simulink model "Exp3_BPSK_mod_demod"  (R2020b)
settings: Solver=VariableStepAuto  StartTime=0.0  StopTime=10.0  RelTol=1e-3
libraries: simulink x3, dspsigops x2, dspstat3 x1, commrandsrc3 x1
settings Model: Creator=Mohit Akhouri  LastModifiedBy=Mohit Akhouri

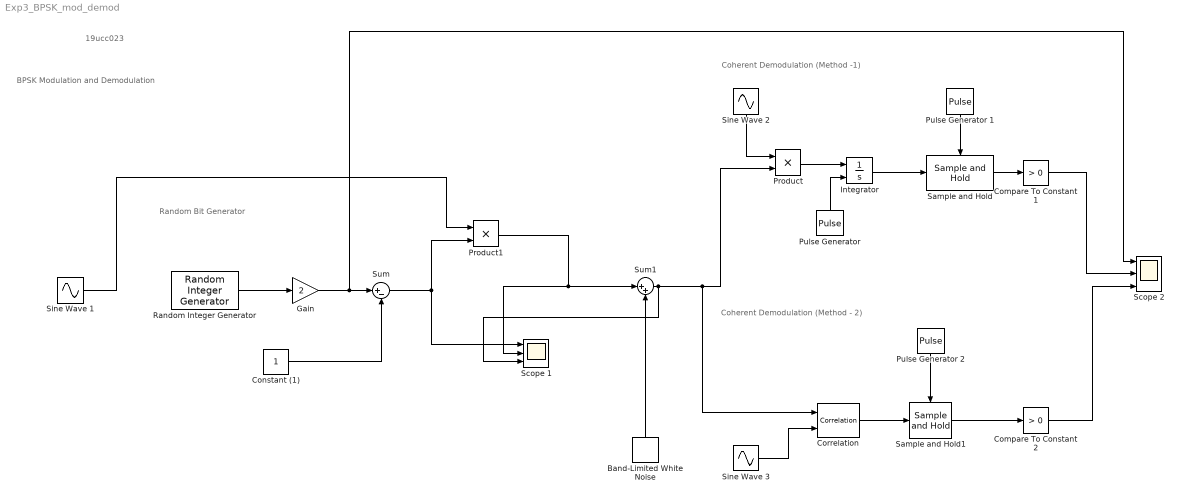
== system Exp3_BPSK_mod_demod ==
  note: BPSK Modulation and Demodulation
  note: 19ucc023
  note: Random Bit Generator
  note: Coherent Demodulation (Method - 2)
  note: Coherent Demodulation (Method -1)
  Band-Limited White Noise : simulink/Sources/Band-Limited White Noise  Cov=[0.0000001]  Ts=0.0001  seed=[23341]
  Compare To Constant 1 : simulink/Logic and Bit Operations/Compare To Constant  relop=>  const=0  OutDataTypeStr=boolean
  Compare To Constant 2 : simulink/Logic and Bit Operations/Compare To Constant  relop=>  const=0  OutDataTypeStr=boolean
  Constant (1) : Constant
  Correlation : dspstat3/Correlation  domain=Time  roundingMode=Floor  overflowMode=off  outputDataTypeStr=Inherit: Same as accumulator  outputMin=[]  outputMax=[]  outputLastDataTypeStr=Inherit: Same as accumulator
      settings: SourceProductBaseCode=DS
  Gain : Gain  Gain=2
  Integrator : Integrator  ExternalReset=rising
  Product : Product
  Product1 : Product
  Pulse Generator : DiscretePulseGenerator  PulseType=Time based  Period=0.5  PulseWidth=50
  Pulse Generator 1 : DiscretePulseGenerator  PulseType=Time based  Period=0.5  PulseWidth=50
  Pulse Generator 2 : DiscretePulseGenerator  PulseType=Time based  Period=0.5  PulseWidth=50
  Random Integer Generator : commrandsrc3/Random Integer Generator  SetSize=2  SeedSource=Auto  Seed=0  SampleTime=0.5  SamplesPerFrame=1  OutputDataType=double  SimulateUsing=Interpreted execution
  Sample and Hold : dspsigops/Sample and Hold  trig=Rising edge  initCond=0  latchinput=on
  Sample and Hold1 : dspsigops/Sample and Hold  trig=Rising edge  initCond=0  latchinput=off
  Scope 1 : Scope  NumInputPorts=3
  Scope 2 : Scope  NumInputPorts=3
  Sine Wave 1 : Sin  Frequency=100  SampleTime=0.5
  Sine Wave 2 : Sin  Frequency=100  SampleTime=0.5
  Sine Wave 3 : Sin  Frequency=100  SampleTime=0.5
  Sum : Sum  Inputs=|+-
  Sum1 : Sum  Inputs=|++
  wires:
  Sine Wave 1/1 -> Product1/1
  Random Integer Generator/1 -> Gain/1
  Gain/1 -> Scope 2/1, Sum/1
  Constant (1)/1 -> Sum/2
  Sum/1 -> Scope 1/1, Product1/2
  Product1/1 -> Scope 1/2, Sum1/1
  Band-Limited White Noise/1 -> Sum1/2
  Sum1/1 -> Scope 1/3, Correlation/1, Product/2
  Sine Wave 3/1 -> Correlation/2
  Sine Wave 2/1 -> Product/1
  Pulse Generator 1/1 -> Sample and Hold/Trigger
  Correlation/1 -> Sample and Hold1/1
  Pulse Generator 2/1 -> Sample and Hold1/Trigger
  Sample and Hold1/1 -> Compare To Constant 2/1
  Compare To Constant 2/1 -> Scope 2/3
  Product/1 -> Integrator/1
  Pulse Generator/1 -> Integrator/2
  Integrator/1 -> Sample and Hold/1
  Sample and Hold/1 -> Compare To Constant 1/1
  Compare To Constant 1/1 -> Scope 2/2
